simulink model "sldemo_hydcyl"  (Simulink 10.0)
settings: Solver=ode45  StartTime=0  StopTime=0.1  RelTol=1e-4  AbsTol=1e-6
model workspace (MATLAB code in the model file):
  | % Load the initial conditions and initialization data
  | % Using the same MAT file as
  | % sldemo_hydcyl
  | % sldemo_hydcyl4
  | % sldemo_hydrod
  | 
  | load sldemo_hydcyl_data;
undefined symbols (not defined in the file): C2, K, Qmax
libraries: hydlib x2
Description:
  | Single Hydraulic Cylinder Simulation
  | 
  | This demo uses Simulink(R) to model a hydraulic cylinder. You can apply these
  | concepts to applications where you need to model hydraulic behavior. See two
  | related demos that use the same basic components:
  | 
  | * four cylinder model: sldemo_hydcyl4
  | * two cylinder model with load constraints: sldemo_hydrod
settings Model: Creator=The MathWorks, Inc.  LastModifiedBy=bhisma  ExtModeTrigMode=oneshot  ExtModeArmWhenConnect=off  ExtModeAutoUpdateStatusClock=off
settings SolverCC: AutoScaleAbsTol=off
settings DataIOCC: SaveOutput=off  SaveTime=off  ReturnWorkspaceOutputs=on  SignalLoggingName=sldemo_hydcyl_output
settings OptimizationCC: BlockReduction=off  BooleanDataType=off  ConditionallyExecuteInputs=off  OptimizeBlockIOStorage=off  BufferReuse=off  GlobalBufferReuse=off  ExpressionFolding=off  ExpressionDepthLimit=2147483647  LocalBlockOutputs=off  InitFltsAndDblsToZero=on  BufferReusableBoundary=off  OptimizeDataStoreBuffers=off  BusAssignmentInplaceUpdate=off
settings DebuggingCC: AlgebraicLoopMsg=none  SaveWithParameterizedLinksMsg=none  SignalResolutionControl=TryResolveAllWithWarning  MultiTaskDSMMsg=warning  MultiTaskCondExecSysMsg=none  SigSpecEnsureSampleTimeMsg=none  IntegerOverflowMsg=none  FcnCallInpInsideContextMsg=warning  BusObjectLabelMismatch=none  StateNameClashWarn=warning  IntegerSaturationMsg=none
settings HardwareCC: TargetUnknown=on
settings GRTTargetCC: TargetFcnLib=ansi_tfl_tmw.mat  GeneratePreprocessorConditionals=Disable all
settings ConfigComp: CovMetricSettings=d  CovExternalEMLEnable=off

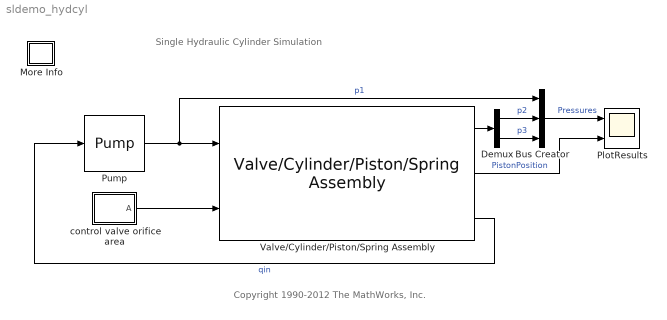
== system sldemo_hydcyl ==
  note: Single Hydraulic Cylinder Simulation
  note: Copyright 1990-2012 The MathWorks, Inc.
  Bus Creator : BusCreator  Inputs=3
  Demux : Demux  Outputs=2
  More Info : Subsystem
      settings: OpenFcn=showExample('simulink_general/sldemo_hydcylExample')
      mask Display: disp('?')
  PlotResults : Scope  NumInputPorts=2
  Pump : hydlib/Pump  t="[0        .04     .04     .05    .05     .1]"  Qpump=Qmax*[1 1 0 0 1 1]  p10=Qmax/C2*2  C2=C2
  Valve/Cylinder/Piston/Spring Assembly : hydlib/Valve//Cylinder//Piston//Spring Assembly  K=K  C1=C1  Ac=Ac  Cd=Cd  rho=rho  V30=V30  beta=Beta  assemblyName=Spring
  control valve orifice area : Subsystem  mask(Ramp){}
      mask Display: plot(0,0,100,100,[98,0],[96,0])
  wires:
  control valve orifice area/1(A) -> Valve/Cylinder/Piston/Spring Assembly/2
  Pump/1 -> Valve/Cylinder/Piston/Spring Assembly/1, Bus Creator/1  "p1"
  Valve/Cylinder/Piston/Spring Assembly/2 -> PlotResults/2  "PistonPosition"
  Valve/Cylinder/Piston/Spring Assembly/3 -> Pump/1  "qin"
  Valve/Cylinder/Piston/Spring Assembly/1 -> Demux/1
  Demux/1 -> Bus Creator/2  "p2"
  Demux/2 -> Bus Creator/3  "p3"
  Bus Creator/1 -> PlotResults/1  "Pressures"

== system sldemo_hydcyl/More Info ==

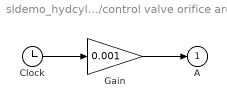
== system sldemo_hydcyl/control valve orifice area ==
  Clock : Clock
  Gain : Gain  Gain=0.001  SaturateOnIntegerOverflow=on  OutDataTypeStr=Inherit: Same as input  ParamDataTypeStr=Inherit: Same as input
  A : Outport  InitialOutput=0  VectorParamsAs1DForOutWhenUnconnected=off
  wires:
  Gain/1 -> A/1
  Clock/1 -> Gain/1
